simulink model "coop_reg_SVFB"  (R2023a)
settings: Solver=VariableStepAuto  StartTime=0.0  StopTime=t_sim  RelTol=1e-3
values from neighbouring files (symbols this model uses):
  A = A_contr    [coop_reg.m]
  B = [0 -9.9453]'    [coop_reg.m]
  C = [708.27 0]    [coop_reg.m]
  D = 0    [coop_reg.m]
  L_obs = place(A',C', [-1 -2])'    [coop_reg.m]
  leader_noise = 0    [coop_reg.m]
  noise_mean = 0    [coop_reg.m]
  noise_seed = randi(100)    [coop_reg.m]
  noise_var = 10    [coop_reg.m]
  x0_0 = x0_0 * x0_ref    [coop_reg.m]
  x0_0_obs = zeros(n,1)    [coop_reg.m]
undefined symbols (not defined in the file or in its folder): coopObserver
libraries: Si_block_2024a x6
settings Model: Creator=federico  LastModifiedBy=Francesco

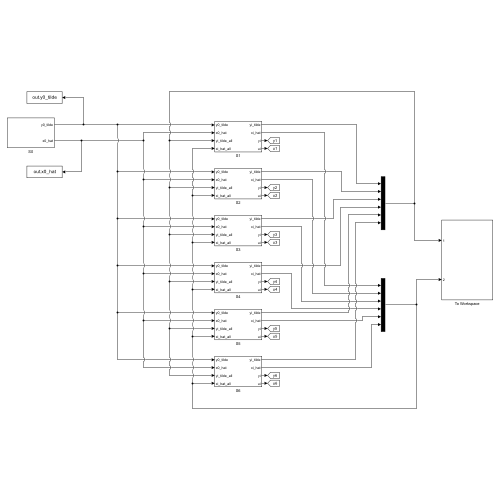
[thumbnail: Simulink's stored preview of the top-level diagram]
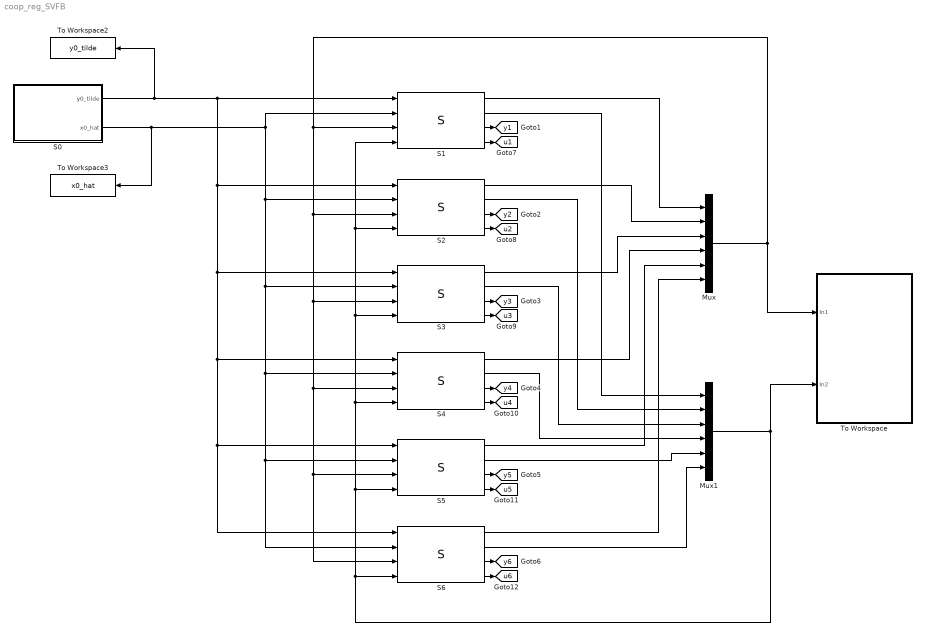
== system coop_reg_SVFB ==
  Mux : Mux  Inputs=6
  Mux1 : Mux  Inputs=6
  S0 : Subsystem
  S1 : Si_block_2024a/S  i=1
  S2 : Si_block_2024a/S  i=2
  S3 : Si_block_2024a/S  i=3
  S4 : Si_block_2024a/S  i=4
  S5 : Si_block_2024a/S  i=5
  S6 : Si_block_2024a/S  i=6
  To Workspace : Subsystem
  To Workspace2 : ToWorkspace  VariableName=y0_tilde  SampleTime=-1
  To Workspace3 : ToWorkspace  VariableName=x0_hat  SampleTime=-1
  tag scope: u1=global, u2=global, u3=global, u4=global, u5=global, u6=global, y1=global, y2=global, y3=global, y4=global, y5=global, y6=global
  wires:
  S1/1 -> Mux/1
  S2/1 -> Mux/2
  S3/1 -> Mux/3
  S4/1 -> Mux/4
  S5/1 -> Mux/5
  S6/1 -> Mux/6
  S1/2 -> Mux1/1
  S2/2 -> Mux1/2
  S3/2 -> Mux1/3
  S4/2 -> Mux1/4
  S5/2 -> Mux1/5
  S6/2 -> Mux1/6
  Mux/1 -> To Workspace/1(In1), S1/3, S2/3, S3/3, S4/3, S6/3, S5/3
  Mux1/1 -> S6/4, S5/4, S4/4, S3/4, S2/4, S1/4, To Workspace/2(In2)
  S0/1(y0_tilde) -> To Workspace2/1, S1/1, S2/1, S3/1, S4/1, S6/1, S5/1
  S0/2(x0_hat) -> To Workspace3/1, S1/2, S2/2, S3/2, S4/2, S6/2, S5/2
  S6/3 -> [y6]
  S5/3 -> [y5]
  S4/3 -> [y4]
  S3/3 -> [y3]
  S2/3 -> [y2]
  S1/3 -> [y1]
  S1/4 -> [u1]
  S2/4 -> [u2]
  S3/4 -> [u3]
  S4/4 -> [u4]
  S5/4 -> [u5]
  S6/4 -> [u6]

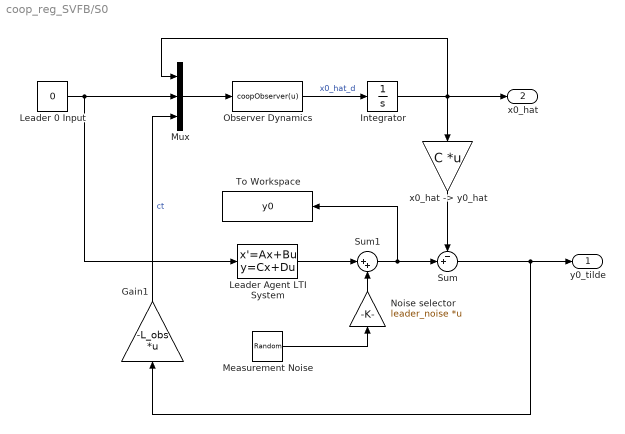
== system coop_reg_SVFB/S0 ==
  Gain1 : Gain  Gain=-L_obs  Multiplication=Matrix(K*u)
  Integrator : Integrator  InitialCondition=x0_0_obs
  Leader 0 Input : Constant  Value=0
  Leader Agent LTI System : StateSpace  A=A  B=B  C=C  D=D  InitialCondition=x0_0
  Measurement Noise : RandomNumber  Mean=noise_mean  Variance=noise_var  Seed=noise_seed  SampleTime=0.1
  Mux : Mux  Inputs=3
  Noise selector : Gain  Gain=leader_noise  Multiplication=Matrix(K*u)
  Observer Dynamics : MATLABFcn  MATLABFcn=coopObserver(u)
  Sum : Sum  Inputs=-+|
  Sum1 : Sum  Inputs=|++
  To Workspace : ToWorkspace  VariableName=y0  SampleTime=-1
  "x0_hat -> y0_hat" : Gain  Gain=C  Multiplication=Matrix(K*u)
  y0_tilde : Outport
  x0_hat : Outport  Port=2
  wires:
  Integrator/1 -> Mux/1, "x0_hat -> y0_hat"/1, x0_hat/1
  Mux/1 -> Observer Dynamics/1
  Observer Dynamics/1 -> Integrator/1  "x0_hat_d"
  Gain1/1 -> Mux/3  "ct"
  Leader 0 Input/1 -> Mux/2, Leader Agent LTI System/1
  Sum/1 -> Gain1/1, y0_tilde/1
  "x0_hat -> y0_hat"/1 -> Sum/1
  Sum1/1 -> To Workspace/1, Sum/2
  Leader Agent LTI System/1 -> Sum1/1
  Noise selector/1 -> Sum1/2
  Measurement Noise/1 -> Noise selector/1

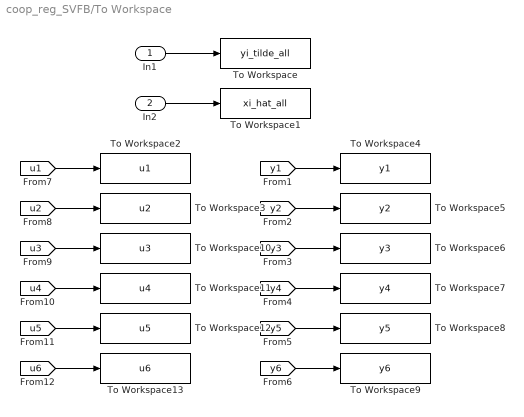
== system coop_reg_SVFB/To Workspace ==
  In1 : Inport
  In2 : Inport  Port=2
  To Workspace : ToWorkspace  VariableName=yi_tilde_all  SampleTime=-1
  To Workspace1 : ToWorkspace  VariableName=xi_hat_all  SampleTime=-1
  To Workspace10 : ToWorkspace  VariableName=u3  SampleTime=-1
  To Workspace11 : ToWorkspace  VariableName=u4  SampleTime=-1
  To Workspace12 : ToWorkspace  VariableName=u5  SampleTime=-1
  To Workspace13 : ToWorkspace  VariableName=u6  SampleTime=-1
  To Workspace2 : ToWorkspace  VariableName=u1  SampleTime=-1
  To Workspace3 : ToWorkspace  VariableName=u2  SampleTime=-1
  To Workspace4 : ToWorkspace  VariableName=y1  SampleTime=-1
  To Workspace5 : ToWorkspace  VariableName=y2  SampleTime=-1
  To Workspace6 : ToWorkspace  VariableName=y3  SampleTime=-1
  To Workspace7 : ToWorkspace  VariableName=y4  SampleTime=-1
  To Workspace8 : ToWorkspace  VariableName=y5  SampleTime=-1
  To Workspace9 : ToWorkspace  VariableName=y6  SampleTime=-1
  wires:
  In1/1 -> To Workspace/1
  In2/1 -> To Workspace1/1
  [y1] -> To Workspace4/1
  [y2] -> To Workspace5/1
  [y5] -> To Workspace8/1
  [y4] -> To Workspace7/1
  [y6] -> To Workspace9/1
  [y3] -> To Workspace6/1
  [u5] -> To Workspace12/1
  [u4] -> To Workspace11/1
  [u1] -> To Workspace2/1
  [u3] -> To Workspace10/1
  [u6] -> To Workspace13/1
  [u2] -> To Workspace3/1
